simulink model "SMDiff"  (R2016b)
settings: Solver=ode4  StartTime=0.0  StopTime=10  FixedStep=1e-5  RelTol=1e-4
values from neighbouring files (symbols this model uses):
  alpha = C + alphaMargin    (= 5)    [DiffSim.m]
  lambda = sqrt(4*C*(alpha + C)/(alpha - C)) + lambdaMargin    [DiffSim.m]
settings Model: Creator=lucac  LastModifiedBy=lucac

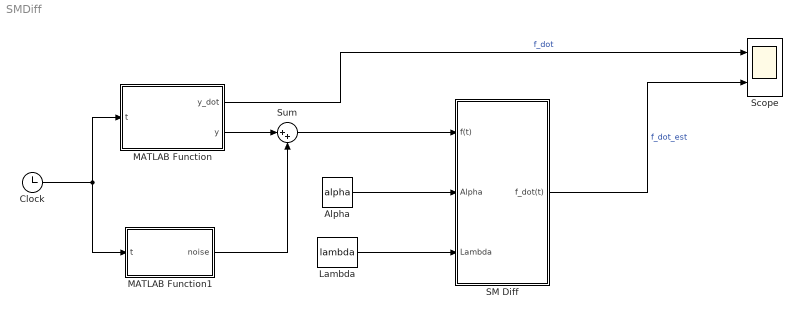
== system SMDiff ==
  Alpha : Constant  Value=alpha
  Clock : Clock
  Lambda : Constant  Value=lambda
  MATLAB Function : MATLAB Function  TreatAsAtomicUnit=on
  MATLAB Function1 : MATLAB Function  TreatAsAtomicUnit=on
  SM Diff : Subsystem
  Scope : Scope  NumInputPorts=2
  Sum : Sum  Inputs=|++
  wires:
  Clock/1 -> MATLAB Function/1(t), MATLAB Function1/1(t)
  Alpha/1 -> SM Diff/2("Alpha ")
  Lambda/1 -> SM Diff/3(Lambda)
  SM Diff/1(f_dot(t)) -> Scope/2  "f_dot_est"
  MATLAB Function/1(y_dot) -> Scope/1  "f_dot"
  MATLAB Function/2(y) -> Sum/1
  Sum/1 -> SM Diff/1(f(t))
  MATLAB Function1/1(noise) -> Sum/2

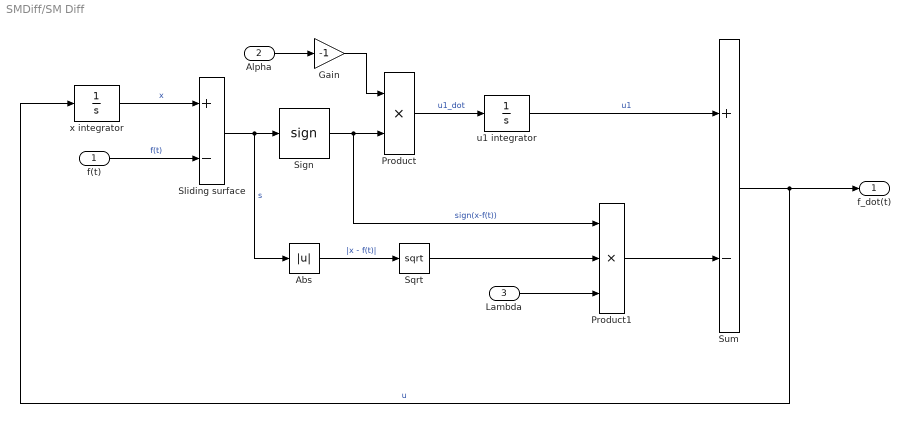
== system SMDiff/SM Diff ==
  f(t) : Inport
  "Alpha " : Inport  Port=2
  Lambda : Inport  Port=3
  Abs : Abs
  Gain : Gain  Gain=-1
  Product : Product
  Product1 : Product  Inputs=3
  Sign : Signum
  Sliding surface : Sum  Inputs=+-
  Sqrt : Sqrt  SaturateOnIntegerOverflow=on
  Sum : Sum  Inputs=+-
  u1 integrator : Integrator
  x integrator : Integrator
  f_dot(t) : Outport
  wires:
  "Alpha "/1 -> Gain/1
  x integrator/1 -> Sliding surface/1  "x"
  f(t)/1 -> Sliding surface/2  "f(t)"
  Sliding surface/1 -> Abs/1, Sign/1  "s"
  Sign/1 -> Product1/1, Product/2  "sign(x-f(t))"
  Gain/1 -> Product/1
  Product/1 -> u1 integrator/1  "u1_dot"
  u1 integrator/1 -> Sum/1  "u1"
  Abs/1 -> Sqrt/1  "|x - f(t)|"
  Sqrt/1 -> Product1/2
  Lambda/1 -> Product1/3
  Product1/1 -> Sum/2
  Sum/1 -> x integrator/1, f_dot(t)/1  "u"

== matlab function SMDiff/MATLAB Function1 ==
  data: t input; noise output
function noise = fcn(t)

noise = 0.001*cos(30*t);

== matlab function SMDiff/MATLAB Function ==
  data: y_dot output; t input; y output
function [y_dot, y] = fcn(t)


y_dot = 3*cos(3*t) + 2*sin(t);
y = sin(3*t) - 2*cos(t);
